simulink model "Complementary_Filter_Simulink"  (R2019b)
settings: Solver=VariableStepAuto  StartTime=0.0  StopTime=15  RelTol=1e-3
undefined symbols (not defined in the file or in its folder): DiscIntNeverNeededParam
libraries: aerolibconvert2 x9
settings Model: Creator=Szabolcs  LastModifiedBy=Szabolcs

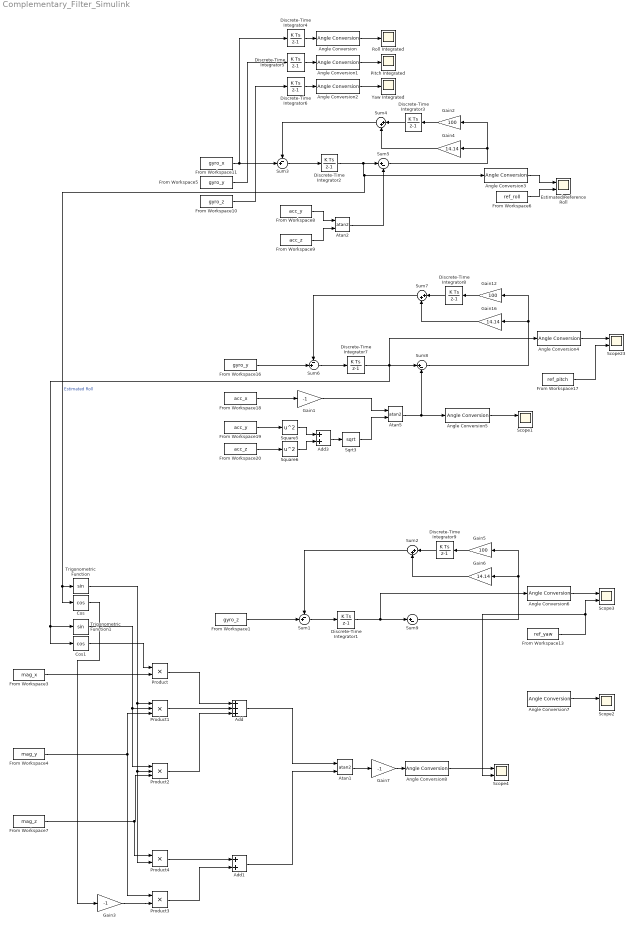
== system Complementary_Filter_Simulink ==
  Add : Sum  Inputs=+++
  Add1 : Sum
  Add3 : Sum
  Angle Conversion{,1..8} (9 alike) : aerolibconvert2/Angle Conversion  IU=rad  OU=deg
  Atan1 : Trigonometry  Operator=atan2
  Atan2 : Trigonometry  Operator=atan2
  Atan5 : Trigonometry  Operator=atan2
  Cos : Trigonometry  Operator=cos
  Cos1 : Trigonometry  Operator=cos
  Discrete-Time Integrator{1,4..9} (7 alike) : DiscreteIntegrator  SampleTime=-1  ICPrevOutput=DiscIntNeverNeededParam  ICPrevScaledInput=DiscIntNeverNeededParam
  Discrete-Time Integrator2 : DiscreteIntegrator  SampleTime=0.01  ICPrevOutput=DiscIntNeverNeededParam  ICPrevScaledInput=DiscIntNeverNeededParam
  Discrete-Time Integrator3 : DiscreteIntegrator  SampleTime=0.01  ICPrevOutput=DiscIntNeverNeededParam  ICPrevScaledInput=DiscIntNeverNeededParam
  Estimated/Reference Roll : Scope  NumInputPorts=2
  From Workspace1 : FromWorkspace  VariableName=gyro_z  SampleTime=0
  From Workspace10 : FromWorkspace  VariableName=gyro_z  SampleTime=0
  From Workspace11 : FromWorkspace  VariableName=gyro_x  SampleTime=0
  From Workspace13 : FromWorkspace  VariableName=ref_yaw  SampleTime=0
  From Workspace16 : FromWorkspace  VariableName=gyro_y  SampleTime=0
  From Workspace17 : FromWorkspace  VariableName=ref_pitch  SampleTime=0
  From Workspace18 : FromWorkspace  VariableName=acc_x  SampleTime=0
  From Workspace19 : FromWorkspace  VariableName=acc_y  SampleTime=0
  From Workspace20 : FromWorkspace  VariableName=acc_z  SampleTime=0
  From Workspace3 : FromWorkspace  VariableName=mag_x  SampleTime=0
  From Workspace4 : FromWorkspace  VariableName=mag_y  SampleTime=0
  From Workspace5 : FromWorkspace  VariableName=gyro_y  SampleTime=0
  From Workspace6 : FromWorkspace  VariableName=ref_roll  SampleTime=0
  From Workspace7 : FromWorkspace  VariableName=mag_z  SampleTime=0
  From Workspace8 : FromWorkspace  VariableName=acc_y  SampleTime=0
  From Workspace9 : FromWorkspace  VariableName=acc_z  SampleTime=0
  Gain1 : Gain  Gain=-1
  Gain12 : Gain  Gain=100
  Gain16 : Gain  Gain=14.14
  Gain2 : Gain  Gain=100
  Gain3 : Gain  Gain=-1
  Gain4 : Gain  Gain=14.14
  Gain5 : Gain  Gain=100
  Gain6 : Gain  Gain=14.14
  Gain7 : Gain  Gain=-1
  Pitch Integrated : Scope
  Product : Product
  Product1 : Product  Inputs=3
  Product2 : Product  Inputs=3
  Product3 : Product
  Product4 : Product
  Roll Integrated : Scope
  Scope{1..4,23} (5 alike) : Scope  NumInputPorts=2
  Sqrt3 : Sqrt  SaturateOnIntegerOverflow=on
  Square5 : Math  Operator=square  SignedPower=off  SaturateOnIntegerOverflow=on
  Square6 : Math  Operator=square  SignedPower=off  SaturateOnIntegerOverflow=on
  Sum1 : Sum  Inputs=-+|
  Sum2 : Sum  Inputs=|++
  Sum3 : Sum  Inputs=-+|
  Sum4 : Sum  Inputs=|++
  Sum5 : Sum  Inputs=|+-
  Sum6 : Sum  Inputs=-+|
  Sum7 : Sum  Inputs=|++
  Sum8 : Sum  Inputs=|+-
  Sum9 : Sum  Inputs=|+-
  Trigonometric Function : Trigonometry
  Trigonometric Function1 : Trigonometry
  Yaw Integrated : Scope
  wires:
  From Workspace5/1 -> Discrete-Time Integrator5/1
  Gain4/1 -> Sum4/2
  Sum5/1 -> Gain4/1, Gain2/1
  Sum4/1 -> Sum3/1
  Sum3/1 -> Discrete-Time Integrator2/1
  Gain2/1 -> Discrete-Time Integrator3/1
  Discrete-Time Integrator2/1 -> Cos/1, Trigonometric Function/1, Angle Conversion3/1, Sum5/1  "Estimated Roll"
  Discrete-Time Integrator3/1 -> Sum4/1
  From Workspace6/1 -> Estimated/Reference Roll/2
  From Workspace11/1 -> Sum3/2, Discrete-Time Integrator4/1
  From Workspace8/1 -> Atan2/1
  From Workspace9/1 -> Atan2/2
  Atan2/1 -> Sum5/2
  From Workspace10/1 -> Discrete-Time Integrator6/1
  Discrete-Time Integrator4/1 -> Angle Conversion/1
  Discrete-Time Integrator5/1 -> Angle Conversion1/1
  Discrete-Time Integrator6/1 -> Angle Conversion2/1
  Angle Conversion3/1 -> Estimated/Reference Roll/1
  Discrete-Time Integrator7/1 -> Trigonometric Function1/1, Cos1/1, Angle Conversion4/1, Sum8/1
  From Workspace17/1 -> Scope23/2
  Gain12/1 -> Discrete-Time Integrator8/1
  From Workspace18/1 -> Gain1/1
  From Workspace19/1 -> Square5/1
  From Workspace20/1 -> Square6/1
  Sum7/1 -> Sum6/1
  From Workspace16/1 -> Sum6/2
  Discrete-Time Integrator8/1 -> Sum7/1
  Sum8/1 -> Gain16/1, Gain12/1
  Gain16/1 -> Sum7/2
  Square6/1 -> Add3/2
  Add3/1 -> Sqrt3/1
  Sqrt3/1 -> Atan5/2
  Square5/1 -> Add3/1
  Atan5/1 -> Angle Conversion5/1, Sum8/2
  Sum6/1 -> Discrete-Time Integrator7/1
  Angle Conversion/1 -> Roll Integrated/1
  Angle Conversion1/1 -> Pitch Integrated/1
  Angle Conversion2/1 -> Yaw Integrated/1
  Angle Conversion4/1 -> Scope23/1
  Angle Conversion5/1 -> Scope1/1
  Gain1/1 -> Atan5/1
  Sum1/1 -> Discrete-Time Integrator1/1
  Discrete-Time Integrator1/1 -> Angle Conversion6/1, Sum9/1
  Gain6/1 -> Sum2/2
  Angle Conversion6/1 -> Scope3/1
  Gain5/1 -> Discrete-Time Integrator9/1
  Angle Conversion7/1 -> Scope2/1
  From Workspace1/1 -> Sum1/2
  Sum2/1 -> Sum1/1
  Discrete-Time Integrator9/1 -> Sum2/1
  Sum9/1 -> Gain6/1, Gain5/1
  From Workspace13/1 -> Scope4/2, Scope3/2
  Cos1/1 -> Product/1
  Trigonometric Function/1 -> Product2/2, Product4/2, Product1/1
  Trigonometric Function1/1 -> Product1/2, Product2/1
  Product/1 -> Add/1
  Product1/1 -> Add/2
  Product2/1 -> Add/3
  Gain3/1 -> Product3/2
  Cos/1 -> Gain3/1
  Product4/1 -> Add1/1
  Product3/1 -> Add1/2
  Atan1/1 -> Gain7/1
  Add1/1 -> Atan1/2
  Add/1 -> Atan1/1
  Gain7/1 -> Angle Conversion8/1
  Angle Conversion8/1 -> Scope4/1
  From Workspace3/1 -> Product/2
  From Workspace4/1 -> Product3/1, Product1/3
  From Workspace7/1 -> Product4/1, Product2/3
